simulink model "Project_Model_0"  (Simulink 7.8)
settings: Solver=ode45  StartTime=0.0  StopTime=10.0  RelTol=1e-3
settings Model: Creator=ipd501  LastModifiedBy=ipd501

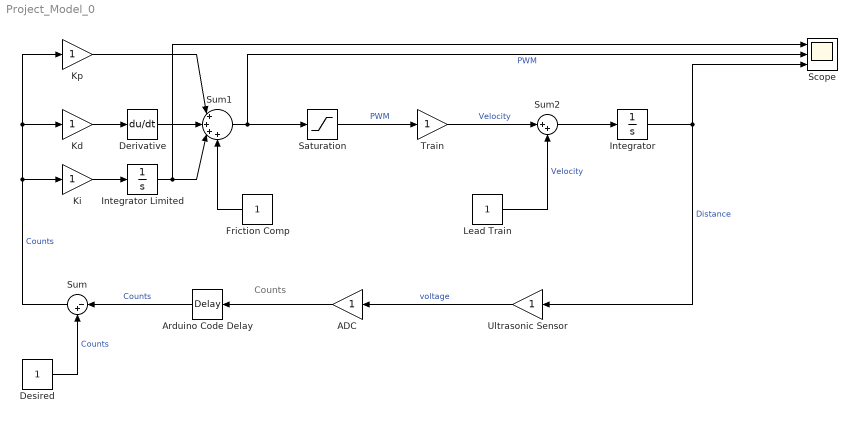
== system Project_Model_0 ==
  note: Counts
  ADC : Gain
  Arduino Code Delay : TransportDelay
  Derivative : Derivative
  Desired : Constant
  Friction Comp : Constant
  Integrator : Integrator
  Integrator Limited : Integrator  LimitOutput=on  UpperSaturationLimit=1  LowerSaturationLimit=0
  Kd : Gain
  Ki : Gain
  Kp : Gain
  Lead Train : Constant
  Saturation : Saturate
  Scope : Scope  NumInputPorts=3
      settings: YMin=-5~-5~-5  YMax=5~5~5
  Sum : Sum  Inputs=|-+
  Sum1 : Sum  Inputs=|++++
  Sum2 : Sum  Inputs=|++
  Train : Gain
  Ultrasonic Sensor : Gain
  wires:
  ADC/1 -> Arduino Code Delay/1
  Desired/1 -> Sum/2  "Counts"
  Arduino Code Delay/1 -> Sum/1  "Counts"
  Kd/1 -> Derivative/1
  Ki/1 -> Integrator Limited/1
  Sum/1 -> Ki/1, Kp/1, Kd/1  "Counts"
  Kp/1 -> Sum1/1
  Derivative/1 -> Sum1/2
  Integrator Limited/1 -> Sum1/3, Scope/1
  Friction Comp/1 -> Sum1/4
  Sum1/1 -> Saturation/1, Scope/2  "PWM"
  Saturation/1 -> Train/1  "PWM"
  Train/1 -> Sum2/1  "Velocity"
  Lead Train/1 -> Sum2/2  "Velocity"
  Sum2/1 -> Integrator/1
  Integrator/1 -> Ultrasonic Sensor/1, Scope/3  "Distance"
  Ultrasonic Sensor/1 -> ADC/1  "voltage"
